simulink model "BANSHEE"  (Simulink 8.1)
settings: Solver=ode1  StartTime=0.0  StopTime=inf  FixedStep=Ts  MaxStep=1e-3  RelTol=1e-3
PostLoadFcn:
  | BANSHEE_init;
InitFcn:
  | BANSHEE_init;
values from neighbouring files (symbols this model uses):
  F1 = xlsread('F1_relay_banshee.xlsx')    [relay_settings_init.m]
  F2 = xlsread('F2_relay_banshee.xlsx')    [relay_settings_init.m]
  F3 = xlsread('F3_relay_banshee.xlsx')    [relay_settings_init.m]
  Ts = 100E-6    (= 0.0001)    [BANSHEE_init.m]    (also in Ghost_init.m)
undefined symbols (not defined in the file or in its folder): Banshee_HWCtrl_IOs, Banshee_SEL751_Woodward_lib, DMS_slave_lib, DMSCommands, fdesignblkfcn, Feeder1_lib, Feeder2_lib, Feeder3_lib, gcbh, generic_ethernet_cb, Hydride, Left, Metal, Nickel, relay_housing_lib, SM_UtilityService, SS_F1_RELAY_HOUSING, SS_F2_RELAY_HOUSING, SS_F3_RELAY_HOUSING, SS_Feeder1, SS_Feeder2, SS_Feeder3, TestSeq_slave_lib, TestSequenceCommands, type, utility_service_lib, V
libraries: powerlib x64, cables_lib x54, breaker_lib x52, rtio_generic_modbus x46, relay_modbus_lib x42, rtio_opalrt_op5142ex1 x37, transformer_lib x29, simulink x26, rteventslib x26, rtlab x24, Load_lib x20, ssn_lib x18
(part 6 of 8)

== system BANSHEE/SM_UtilityService/Banshee_HWCtrl_IOs/Woodward Inputs ==
  note: Copyright (c) 2016 Massachusetts Institute of Technology
      | Permission is hereby granted, free of charge, to any person obtaining a copy of this software and associated documentation files (the "Software"), to deal
      | in the Software without restriction, including without limitation the rights to use, copy, modify, merge, publish, distribute, sublicense, and/or sell copies of the
      | Software, and to permit persons to whom the Software is furnished to do so, subject to the following conditions:
      |
      | THE SOFTWARE IS PROVIDED "AS IS", WITHOUT WARRANTY OF ANY KIND, EXPRESS OR IMPLIED, INCLUDING BUT NOT LIMITED TO THE
      | WARRANTIES OF MERCHANTABILITY, FITNESS FOR A PARTICULAR PURPOSE AND NONINFRINGEMENT. IN NO EVENT SHALL THE AUTHORS
      | OR COPYRIGHT HOLDERS BE LIABLE FOR ANY CLAIM, DAMAGES OR OTHER LIABILITY, WHETHER IN AN ACTION OF CONTRACT, TORT OR
      | OTHERWISE, ARISING FROM, OUT OF OR IN CONNECTION WITH THE SOFTWARE OR THE USE OR OTHER DEALINGS IN THE SOFTWARE
  note: GR1 A AOUT (CH00-15)
  note: All signals should be scaled accordingly prior connecting to this block
  Generator1_Voltage : Inport
  Generator1_Current : Inport  Port=2
  Mains1_Voltage : Inport  Port=3
  Mains1_Current : Inport  Port=4
  MPU1_speed : Inport  Port=5
  Generator2_Voltage : Inport  Port=6
  Generator2_Current : Inport  Port=7
  Mains2_Voltage : Inport  Port=8
  Mains2_Current : Inport  Port=9
  MPU2_speed : Inport  Port=10
  AnalogOut : rtio_opalrt_common/AnalogOut  CtrlName='OpCtrl'  portNb=1  FcnNos=Slot 1 Module A Subsection 1  size=16  maxcount=8  count=8  numchan=8  israngeinput=off  voltagerange=[-16 ... 16]  slot=0  side=0  mismatch=0  slotside=Slot_1_Module_A
      settings: AttributesFormatString=%<CtrlName>
  AnalogOut1 : rtio_opalrt_common/AnalogOut  CtrlName='OpCtrl'  portNb=2  FcnNos=Slot 1 Module A Subsection 2  size=16  maxcount=8  count=8  numchan=8  israngeinput=off  voltagerange=[-16 ... 16]  slot=0  side=0  mismatch=0  slotside=Slot_1_Module_A
      settings: AttributesFormatString=%<CtrlName>
  AnalogOut2 : rtio_opalrt_common/AnalogOut  CtrlName='OpCtrl'  portNb=3  FcnNos=Slot 2 Module A Subsection 1  size=16  maxcount=8  count=8  numchan=8  israngeinput=off  voltagerange=[-16 ... 16]  slot=1  side=0  mismatch=0  slotside=Slot_2_Module_A
      settings: AttributesFormatString=%<CtrlName>
  AnalogOut3 : rtio_opalrt_common/AnalogOut  CtrlName='OpCtrl'  portNb=4  FcnNos=Slot 2 Module A Subsection 2  size=16  maxcount=8  count=8  numchan=8  israngeinput=off  voltagerange=[-16 ... 16]  slot=1  side=0  mismatch=0  slotside=Slot_2_Module_A
      settings: AttributesFormatString=%<CtrlName>
  Demux : Demux  Outputs=2
  Demux{1..5,7..9} (8 alike) : Demux  Outputs=3
  Demux6 : Demux  Outputs=2
  Mux{,1,3..4} (4 alike) : Mux  Inputs=8
  Mux2 : Mux  Inputs=2
  Mux5 : Mux  Inputs=2
  Terminator{,1..3} (4 alike) : Terminator
  wires:
  Mains1_Voltage/1 -> Demux2/1
  Generator1_Voltage/1 -> Demux1/1
  Mux2/1 -> Demux/1
  Mux1/1 -> Mux2/2
  Mux/1 -> Mux2/1
  Demux/2 -> AnalogOut1/1
  Demux/1 -> AnalogOut/1
  AnalogOut1/1 -> Terminator1/1
  AnalogOut/1 -> Terminator/1
  Demux1/1 -> Mux/1
  Demux1/2 -> Mux/2
  Demux1/3 -> Mux/3
  Demux2/1 -> Mux/4
  Demux2/2 -> Mux/5
  Demux2/3 -> Mux/6
  MPU1_speed/1 -> Mux1/5
  Demux4/1 -> Mux/7
  Demux4/2 -> Mux/8
  Demux4/3 -> Mux1/1
  Demux5/1 -> Mux1/2
  Demux5/2 -> Mux1/3
  Demux5/3 -> Mux1/4
  Mux5/1 -> Demux6/1
  Mux4/1 -> Mux5/2
  Mux3/1 -> Mux5/1
  Demux6/2 -> AnalogOut3/1
  Demux6/1 -> AnalogOut2/1
  AnalogOut3/1 -> Terminator3/1
  AnalogOut2/1 -> Terminator2/1
  Generator1_Current/1 -> Demux3/1
  Demux3/1 -> Mux3/2
  Demux3/2 -> Mux3/3
  Demux3/3 -> Mux3/4
  Mains1_Current/1 -> Demux7/1
  Demux7/1 -> Mux3/1
  Mains2_Voltage/1 -> Demux5/1
  Generator2_Voltage/1 -> Demux4/1
  MPU2_speed/1 -> Mux1/6
  Mains2_Current/1 -> Demux8/1
  Demux8/1 -> Mux3/5
  Generator2_Current/1 -> Demux9/1
  Demux9/1 -> Mux3/6
  Demux9/2 -> Mux3/7
  Demux9/3 -> Mux3/8

== system BANSHEE/SM_UtilityService/Banshee_HWCtrl_IOs/Woodward Outputs - Diesel - Gen2 ==
  note: Copyright (c) 2016 Massachusetts Institute of Technology
      | Permission is hereby granted, free of charge, to any person obtaining a copy of this software and associated documentation files (the "Software"), to deal
      | in the Software without restriction, including without limitation the rights to use, copy, modify, merge, publish, distribute, sublicense, and/or sell copies of the
      | Software, and to permit persons to whom the Software is furnished to do so, subject to the following conditions:
      |
      | THE SOFTWARE IS PROVIDED "AS IS", WITHOUT WARRANTY OF ANY KIND, EXPRESS OR IMPLIED, INCLUDING BUT NOT LIMITED TO THE
      | WARRANTIES OF MERCHANTABILITY, FITNESS FOR A PARTICULAR PURPOSE AND NONINFRINGEMENT. IN NO EVENT SHALL THE AUTHORS
      | OR COPYRIGHT HOLDERS BE LIABLE FOR ANY CLAIM, DAMAGES OR OTHER LIABILITY, WHETHER IN AN ACTION OF CONTRACT, TORT OR
      | OTHERWISE, ARISING FROM, OUT OF OR IN CONNECTION WITH THE SOFTWARE OR THE USE OR OTHER DEALINGS IN THE SOFTWARE
  Gen2 MCB Status : Inport
  WoodwardBias : Inport  Port=2
  Bus Creator1 : BusCreator  Inputs=1
  DIO - Gr3 : Subsystem
  DIO - Woodward : Subsystem
  DOUT type config : Subsystem
  Woodward Primary Inputs - Gen2 : Subsystem
  Digital Inputs : Outport
  Gen2 Gov and AVR : Outport  Port=2
  Gen2 Fuel Enable : Outport  Port=3
  Gen2 GCB : Outport  Port=4
  Gen2 MCB : Outport  Port=5
  wires:
  Bus Creator1/1 -> Digital Inputs/1
  DIO - Woodward/1(DIn1) -> DIO - Gr3/1(Dout)
  DIO - Gr3/1(DIn) -> Bus Creator1/1, DIO - Woodward/1(Din_Wood)  "DIN"
  Woodward Primary Inputs - Gen2/1(Gen2 Gov and AVR) -> Gen2 Gov and AVR/1
  DIO - Woodward/3(Gen2 GCB) -> Gen2 GCB/1
  DIO - Woodward/2(Gen2 Fuel Enable) -> Gen2 Fuel Enable/1
  DIO - Woodward/4(Gen2 MCB) -> Gen2 MCB/1
  Gen2 MCB Status/1 -> DIO - Woodward/2(Gen2 MCB Status)
  WoodwardBias/1 -> Woodward Primary Inputs - Gen2/1(WoodwardBias)

== system BANSHEE/SM_UtilityService/Banshee_HWCtrl_IOs/Woodward Outputs - NGCHP - Gen1 ==
  note: Copyright (c) 2016 Massachusetts Institute of Technology
      | Permission is hereby granted, free of charge, to any person obtaining a copy of this software and associated documentation files (the "Software"), to deal
      | in the Software without restriction, including without limitation the rights to use, copy, modify, merge, publish, distribute, sublicense, and/or sell copies of the
      | Software, and to permit persons to whom the Software is furnished to do so, subject to the following conditions:
      |
      | THE SOFTWARE IS PROVIDED "AS IS", WITHOUT WARRANTY OF ANY KIND, EXPRESS OR IMPLIED, INCLUDING BUT NOT LIMITED TO THE
      | WARRANTIES OF MERCHANTABILITY, FITNESS FOR A PARTICULAR PURPOSE AND NONINFRINGEMENT. IN NO EVENT SHALL THE AUTHORS
      | OR COPYRIGHT HOLDERS BE LIABLE FOR ANY CLAIM, DAMAGES OR OTHER LIABILITY, WHETHER IN AN ACTION OF CONTRACT, TORT OR
      | OTHERWISE, ARISING FROM, OUT OF OR IN CONNECTION WITH THE SOFTWARE OR THE USE OR OTHER DEALINGS IN THE SOFTWARE
  Gen1 MCB Status : Inport
  WoodwardBias : Inport  Port=2
  Bus Creator1 : BusCreator  Inputs=1
  DIO - Gr3 : Subsystem
  DIO - Woodward : Subsystem
  DOUT type config : Subsystem
  Woodward Primary Inputs - Gen1 : Subsystem
  Digital Inputs : Outport
  Gen1 Gov and AVR : Outport  Port=2
  Gen1 Fuel Enable : Outport  Port=3
  Gen1 GCB : Outport  Port=4
  Gen1 MCB : Outport  Port=5
  wires:
  DIO - Woodward/4(DIn1) -> DIO - Gr3/1(Dout)
  DIO - Gr3/1(DIn) -> DIO - Woodward/1(Din_Wood), Bus Creator1/1  "DIN"
  Bus Creator1/1 -> Digital Inputs/1
  Woodward Primary Inputs - Gen1/1(Gen1 Gov and AVR) -> Gen1 Gov and AVR/1
  WoodwardBias/1 -> Woodward Primary Inputs - Gen1/1(WoodwardBias)
  DIO - Woodward/2(Gen1 GCB) -> Gen1 GCB/1
  DIO - Woodward/3(Gen1 MCB) -> Gen1 MCB/1
  DIO - Woodward/1(Gen1 Fuel Enable) -> Gen1 Fuel Enable/1
  Gen1 MCB Status/1 -> DIO - Woodward/2(Gen1 MCB Status)

== system BANSHEE/SM_UtilityService/DataSet_Diesel_CHP_PCCs/Status ==
  SEL751 : Inport
  CBX03 : Inport  Port=2
  GCB : Inport  Port=3
  Data Type Conversion{,1..3} (4 alike) : DataTypeConversion
  Gain : Gain  Gain=2
  Gain1 : Gain  Gain=4
  Sum : Sum  Inputs=+++
  o : Outport
  wires:
  GCB/1 -> Data Type Conversion2/1
  CBX03/1 -> Data Type Conversion1/1
  SEL751/1 -> Data Type Conversion/1
  Gain/1 -> Sum/2
  Gain1/1 -> Sum/3
  Sum/1 -> Data Type Conversion3/1
  Data Type Conversion/1 -> Sum/1
  Data Type Conversion1/1 -> Gain/1
  Data Type Conversion2/1 -> Gain1/1
  Data Type Conversion3/1 -> o/1

== system BANSHEE/SM_UtilityService/DataSet_Diesel_CHP_PCCs/Status1 ==
  SEL751 : Inport
  CBX03 : Inport  Port=2
  GCB : Inport  Port=3
  Data Type Conversion{,1..3} (4 alike) : DataTypeConversion
  Gain : Gain  Gain=2
  Gain1 : Gain  Gain=4
  Sum : Sum  Inputs=+++
  o : Outport
  wires:
  GCB/1 -> Data Type Conversion2/1
  CBX03/1 -> Data Type Conversion1/1
  SEL751/1 -> Data Type Conversion/1
  Gain/1 -> Sum/2
  Gain1/1 -> Sum/3
  Sum/1 -> Data Type Conversion3/1
  Data Type Conversion/1 -> Sum/1
  Data Type Conversion1/1 -> Gain/1
  Data Type Conversion2/1 -> Gain1/1
  Data Type Conversion3/1 -> o/1

== system BANSHEE/SM_UtilityService/Number of seconds of recording/Increment ==
  Trigger : TriggerPort
  Increment : Constant
  Memory : Memory  InheritSampleTime=on
  Sum : Sum  Inputs=|++
  Out1 : Outport
  wires:
  Increment/1 -> Sum/2
  Memory/1 -> Sum/1
  Sum/1 -> Memory/1, Out1/1

== system BANSHEE/SM_UtilityService/Number of seconds of recording1/Increment ==
  Trigger : TriggerPort
  Increment : Constant
  Memory : Memory  InheritSampleTime=on
  Sum : Sum  Inputs=|++
  Out1 : Outport
  wires:
  Increment/1 -> Sum/2
  Memory/1 -> Sum/1
  Sum/1 -> Memory/1, Out1/1

== system BANSHEE/SM_UtilityService/selected_Irms_a/rms_a ==
  i : Inport
  Demux1 : Demux  Outputs=3
  RMS_Calculator : RMS_lib/RMS_Calculator  Ts=Ts
  Terminator8 : Terminator
  Terminator9 : Terminator
  o : Outport
  wires:
  i/1 -> Demux1/1
  RMS_Calculator/1 -> o/1
  Demux1/1 -> RMS_Calculator/1
  Demux1/2 -> Terminator8/1
  Demux1/3 -> Terminator9/1

== system BANSHEE/SM_UtilityService/selected_Irms_a/rms_a1 ==
  i : Inport
  Demux1 : Demux  Outputs=3
  RMS_Calculator : RMS_lib/RMS_Calculator  Ts=Ts
  Terminator8 : Terminator
  Terminator9 : Terminator
  o : Outport
  wires:
  i/1 -> Demux1/1
  RMS_Calculator/1 -> o/1
  Demux1/1 -> RMS_Calculator/1
  Demux1/2 -> Terminator8/1
  Demux1/3 -> Terminator9/1

== system BANSHEE/SM_UtilityService/selected_Irms_a/rms_a2 ==
  i : Inport
  Demux1 : Demux  Outputs=3
  RMS_Calculator : RMS_lib/RMS_Calculator  Ts=Ts
  Terminator8 : Terminator
  Terminator9 : Terminator
  o : Outport
  wires:
  i/1 -> Demux1/1
  RMS_Calculator/1 -> o/1
  Demux1/1 -> RMS_Calculator/1
  Demux1/2 -> Terminator8/1
  Demux1/3 -> Terminator9/1

== system BANSHEE/SM_UtilityService/selected_Irms_a/rms_a3 ==
  i : Inport
  Demux1 : Demux  Outputs=3
  RMS_Calculator : RMS_lib/RMS_Calculator  Ts=Ts
  Terminator8 : Terminator
  Terminator9 : Terminator
  o : Outport
  wires:
  i/1 -> Demux1/1
  RMS_Calculator/1 -> o/1
  Demux1/1 -> RMS_Calculator/1
  Demux1/2 -> Terminator8/1
  Demux1/3 -> Terminator9/1

== system BANSHEE/SM_UtilityService/selected_Irms_a/rms_a4 ==
  i : Inport
  Demux1 : Demux  Outputs=3
  RMS_Calculator : RMS_lib/RMS_Calculator  Ts=Ts
  Terminator8 : Terminator
  Terminator9 : Terminator
  o : Outport
  wires:
  i/1 -> Demux1/1
  RMS_Calculator/1 -> o/1
  Demux1/1 -> RMS_Calculator/1
  Demux1/2 -> Terminator8/1
  Demux1/3 -> Terminator9/1

== system BANSHEE/SM_UtilityService/selected_Irms_a/rms_a5 ==
  i : Inport
  Demux1 : Demux  Outputs=3
  RMS_Calculator : RMS_lib/RMS_Calculator  Ts=Ts
  Terminator8 : Terminator
  Terminator9 : Terminator
  o : Outport
  wires:
  i/1 -> Demux1/1
  RMS_Calculator/1 -> o/1
  Demux1/1 -> RMS_Calculator/1
  Demux1/2 -> Terminator8/1
  Demux1/3 -> Terminator9/1

== system BANSHEE/SM_UtilityService/selected_Irms_a/rms_a6 ==
  i : Inport
  Demux1 : Demux  Outputs=3
  RMS_Calculator : RMS_lib/RMS_Calculator  Ts=Ts
  Terminator8 : Terminator
  Terminator9 : Terminator
  o : Outport
  wires:
  i/1 -> Demux1/1
  RMS_Calculator/1 -> o/1
  Demux1/1 -> RMS_Calculator/1
  Demux1/2 -> Terminator8/1
  Demux1/3 -> Terminator9/1

== system BANSHEE/SM_UtilityService/selected_Irms_a/rms_a7 ==
  i : Inport
  Demux1 : Demux  Outputs=3
  RMS_Calculator : RMS_lib/RMS_Calculator  Ts=Ts
  Terminator8 : Terminator
  Terminator9 : Terminator
  o : Outport
  wires:
  i/1 -> Demux1/1
  RMS_Calculator/1 -> o/1
  Demux1/1 -> RMS_Calculator/1
  Demux1/2 -> Terminator8/1
  Demux1/3 -> Terminator9/1

== system BANSHEE/SM_UtilityService/selected_Irms_a/rms_a8 ==
  i : Inport
  Demux1 : Demux  Outputs=3
  RMS_Calculator : RMS_lib/RMS_Calculator  Ts=Ts
  Terminator8 : Terminator
  Terminator9 : Terminator
  o : Outport
  wires:
  i/1 -> Demux1/1
  RMS_Calculator/1 -> o/1
  Demux1/1 -> RMS_Calculator/1
  Demux1/2 -> Terminator8/1
  Demux1/3 -> Terminator9/1

== system BANSHEE/SM_UtilityService/selected_Irms_a/rms_a9 ==
  i : Inport
  Demux1 : Demux  Outputs=3
  RMS_Calculator : RMS_lib/RMS_Calculator  Ts=Ts
  Terminator8 : Terminator
  Terminator9 : Terminator
  o : Outport
  wires:
  i/1 -> Demux1/1
  RMS_Calculator/1 -> o/1
  Demux1/1 -> RMS_Calculator/1
  Demux1/2 -> Terminator8/1
  Demux1/3 -> Terminator9/1

== system BANSHEE/SS_F3_RELAY_HOUSING/Banshee UDP Data - Formatted Packets/Ethernet communication interface ==
  note: Ethernet communication interface example model
  Data trigger : Inport
  Data to send : Inport  Port=2
  AsyncEthernetCtrl : S-Function  InitFcn=generic_ethernet_cb('initfcn');  FunctionName=sfun_gen_async_ctrl  Parameters=ctrl_id, nbr_to_remote_endpoint, type_to_remote_endpoint,nbr_from_remote_endpoint,type_from_remote_endpoint,protocol,tcp_mode, port, offset_to_remote_endpoint,offset_from_remote_endpoint,swap_tx,swap_rx,0,nic_name,remote_ip,'','','','','','','','','','',exe_name,0  EnableBusSupport=off  mask(AsyncEthernetCtrl){ctrl_id=1, nbr_to_remote_endpoint=342, type_to_remote_endpoint=INT32, offset_to_remote_endpoint=0, nbr_from_remote_endpoint=4, type_from_remote_endpoint=DOUBLE, offset_from_remote_endpoint=0, nic_name=eth0, protocol=UDP, tcp_mode=Server, port=7200, remote_ip=255.255.255.255, exe_name=AsyncEthernet, swap_tx=off, swap_rx=off}
      mask prompts: ctrl_id "Controller ID"; nbr_to_remote_endpoint "Number of data to send"; type_to_remote_endpoint "Type of data to send"; offset_to_remote_endpoint "Byte offset of transmission buffer"; nbr_from_remote_endpoint "Number of data expected to be received"; type_from_remote_endpoint "Type of data expected to be received"; offset_from_remote_endpoint "Byte offset of reception buffer"; nic_name "Network interface name"; tcp_mode "TCP mode"; remote_ip "Remote IP address"; exe_name "Name of the executable"; swap_tx "Swap data endianness before transmission"; swap_rx "Swap data endianness after reception"
      mask help: Generic asynchronous process configuration block
      mask Help: eval('rtlab_help(''opasyncgenctrl'');');
      mask TypeOptions type_to_remote_endpoint: UINT8 | INT8 | UINT16 | INT16 | UINT32 | INT32 | FLOAT | DOUBLE
      mask TypeOptions type_from_remote_endpoint: UINT8 | INT8 | UINT16 | INT16 | UINT32 | INT32 | FLOAT | DOUBLE
      mask TypeOptions protocol: UDP | TCP
      mask TypeOptions tcp_mode: Client | Server
      mask Display: disp(sprintf('\nEthernet communication \ninterface controller\n'))
  B-width : SignalSpecification  Dimensions=nbr_from_remote_endpoint
  Constant : Constant  Value=1000
  Logo : opal_lib/Logo1  vide=[]
  Mux : Mux  Inputs=2
  OpAsyncRecv : rtlab/Communication/Asynchronous/OpAsyncRecv  ctl_id=ctrl_id  recv_id=ctrl_id  enable_param=off  fp1=1  fp2=2  fp3=3  fp4=4  fp5=5  sp1=string1  sp2=string2  sp3=string3  sp4=string4  sp5=string5
  OpAsyncSend : rtlab/Communication/Asynchronous/OpAsyncSend  ctl_id=ctrl_id  send_id=ctrl_id  mode=DONT_NEED_REPLY  enable_param=off  fp1=1  fp2=2  fp3=3  fp4=4  fp5=5  sp1=string1  sp2=string2  sp3=string3  sp4=string4  sp5=string5
  Terminator : Terminator
  Data received : Outport
  Status : Outport  Port=2
  wires:
  Data to send/1 -> OpAsyncSend/2
  Data trigger/1 -> OpAsyncSend/1
  OpAsyncSend/1 -> Mux/1
  OpAsyncRecv/1 -> Mux/2
  Mux/1 -> Status/1
  Constant/1 -> OpAsyncRecv/1
  OpAsyncRecv/2 -> Terminator/1
  OpAsyncRecv/3 -> B-width/1
  B-width/1 -> Data received/1

== system BANSHEE/SS_PV_BESS/EPC/BMS_Modbus ==
  BESS_MS : Inport
  Bus Selector : BusSelector  OutputSignals=Battery_Meas.SOC (%),Battery_Meas.Current (A),Battery_Meas.Voltage (V),BESS_MX1.cb_ms.Status,BESS_MX1.VRMSLL,BESS_MX1.Freq,BESS_MX1.kw,BESS_MX1.kvar
  Gain : Gain  Gain=100
  Gain1 : Gain  Gain=100
  Modbus device6 : rtio_generic_modbus/Modbus device  conf_name=EPC_BMS_cfg.opal  conf_name_mask=EPC_BMS_cfg.xls  sample_time=Ts
  Mux : Mux  Inputs=8
  wires:
  Bus Selector/7 -> Mux/7  "<kw>"
  Bus Selector/5 -> Mux/5  "<VRMSLL>"
  Bus Selector/1 -> Gain/1  "<SOC (%)>"
  Bus Selector/6 -> Gain1/1  "<Freq>"
  Bus Selector/8 -> Mux/8  "<kvar>"
  BESS_MS/1 -> Bus Selector/1
  Gain/1 -> Mux/1
  Bus Selector/3 -> Mux/3  "<Voltage (V)>"
  Bus Selector/2 -> Mux/2  "<Current (A)>"
  Bus Selector/4 -> Mux/4  "<Status>"
  Gain1/1 -> Mux/6
  Mux/1 -> Modbus device6/1

== system BANSHEE/SS_PV_BESS/EPC/Contactors1 ==
  note: with 10ohm resistor
  note: changed to 1000
      | to slow down the time
  Precharge : Inport
  Main Contactor : Inport  Port=2
  Brk_Battery : powerlib/Power Electronics/Ideal Switch  Ron=0.001  Lon=0  IC=0  Rs=1e6  Cs=inf  Measurements=on
  Brk_Precharge : powerlib/Power Electronics/Ideal Switch  Ron=1  Lon=0  IC=0  Rs=1e6  Cs=inf  Measurements=on
  DC+ Source : PMIOPort  Port=1  Side=Right
  DC+ Bus : PMIOPort  Port=2  Side=Left
  DC- Source : PMIOPort  Port=3  Side=Left
  DC- Bus : PMIOPort  Port=4  Side=Right
  wires:
  Precharge/1 -> Brk_Precharge/1
  Main Contactor/1 -> Brk_Battery/1
  connections:
  Brk_Battery/LConn1 -- DC+ Bus/RConn1 -- Brk_Precharge/LConn1
  Brk_Battery/RConn1 -- DC+ Source/RConn1 -- Brk_Precharge/RConn1
  DC- Bus/RConn1 -- DC- Source/RConn1

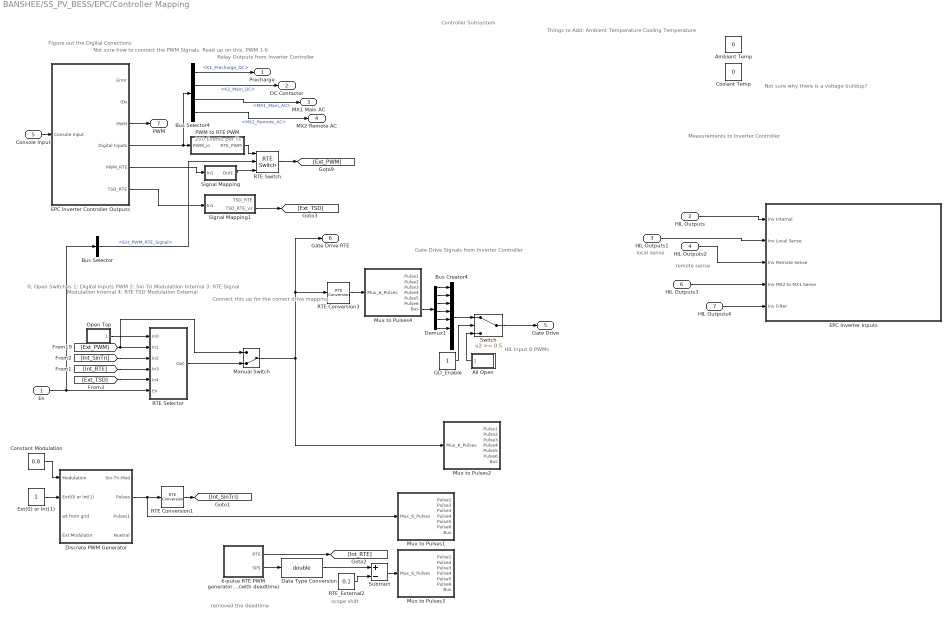
== system BANSHEE/SS_PV_BESS/EPC/Controller Mapping ==
  note: Controller Subsystem
  note: Gate Drive Signals from
      | Inverter Controller
  note: Relay Outputs from
      | Inverter Controller
  note: Measurements to
      | Inverter Controller
  note: Not sure why there is a voltage buildup?
  note: Things to Add:
      | Ambient Temperature
      | Cooling Temperature
  note: HIL Input
      | 8 PWMs
  note: local sense
  note: remote sense
  note: Not sure how to connect
      | the PWM Signals.
      | Read up on this.
      | PWM 1-6
  note: Figure out the
      | Digital Conections
  note: removed the deadtime
  note: scope shift
  note: 0; Open Switches
      | 1: Digital Inputs PWM
      | 2: Sin Tri Modulatiion Internal
      | 3: RTE Signal Modulation Internal
      | 4: RTE TSD Modulation External
  note: 200 Events per Ts
  note: Connect this
      | up for the
      | correct drive
      | mapping.
  En : Inport
  HIL Outputs : Inport  Port=2
  HIL Outputs1 : Inport  Port=3
  HIL Outputs2 : Inport  Port=4
  Console Input : Inport  Port=5
  HIL Outputs3 : Inport  Port=6
  HIL Outputs4 : Inport  Port=7
  6-pulse RTE PWM generator (with deadtime) : Subsystem  Tag=RTEcontrol_s38shd7k88  AncestorBlock=|  mask(3-phase RT-Event Discrete PWM Generator){GeneratorMode=3-arm  bridge (6 pulses), Fc=5000, Ts=Ts, mIndex=0.9, Freq=60, Phase=0, Tdead=0}
      | artemis/Tools /Rt-Event 
      | control blocks/6-pulse RTE
      | PWM generator
      | (with deadtime)
      mask prompts: GeneratorMode "Generator Mode"; Fc "Carrier frequency (Hz):"; Ts "Sample time:"; mIndex "Modulation index  (0<m<1) :"; Freq "Frequency of output voltage (Hz)"; Phase "Phase of output voltage (degrees)"; Tdead "Deadtime (s)"
      mask help:
      | This  block generates RT-Event pulses for 3-phase discrete time compensated  carrier-based PWM (Pulse Width Modulation), self-commutated IGBTs,GTOs or FETs bridges in ARTEMIS-RTE.
      |
      | RT-Event pulses are pair of signals that contain the logical value of the switch {on.off} and a timing value used in ARTEMIS-RTE to compensate for in-step switching actions.
      | PSB pulses consist of the logicla part only.
      |
      | Pulses 1,3 and 5 are respectively for the upper switches of the first,second and third arm. Pulses 2,4 and 6 are for the lower switches.
      mask init:
      | set_param(gcb,'LinkStatus','inactive');
      | if Freq==0
      |     Phase=90;
      | end
      |     Internal_Phase=[0 -2*pi/3 2*pi/3];
      |     Signal_PortWidth=3;
      |     Select1_Elements=[1 4 2 5 3 6];
      |     Select1_PortWidth=6;
      |    Select3_Elements=[1 2 3 4 5 6];
      |    Select3_PortWidth=12;
      mask TypeOptions GeneratorMode: 3-arm  bridge (6 pulses)
      mask Display: plot(0,0,100,100,[60,57,57,56,56,53,53,50,50,47,47,41,41,38,38,35,35,32,32,31,31,25,25,24,24,22,22,19,19,16,16,11,11,8,8,5,5,3,3,2,2,0],[20,20,80,80,20,20,80,80,20,20,80,80,20,20,80,80,20,20,80,80,20,20,80,80,20,20,80,80,20,20,80,80,20,20,80,80,20,20,80,80,20,20])
  All Open : Subsystem
  Ambient Temp : Constant  Value=0
  Bus Creator4 : BusCreator  Inputs=8
  Bus Selector : BusSelector  OutputSignals=Ext_PWM_RTE_Signal
  Bus Selector4 : BusSelector  OutputSignals=DIN.DI_CH00-07.K1_Precharge_DC,DIN.DI_CH00-07.K2_Main_DC,DIN.DI_CH00-07.MX1_Main_AC,DIN.DI_CH00-07.MX2_Remote_AC
  Constant Modulation : Constant  Value=0.8
  Coolant Temp : Constant  Value=0
  Data Type Conversion : DataTypeConversion  OutDataTypeStr=double
  Demux1 : Demux  Outputs=6
  Discrete PWM Generator : Subsystem  AncestorBlock=|  DialogController=POWERSYS.PowerSysDialog  mask(Discrete PWM Generator){GeneratorMode=3-arm  bridge (6 pulses), Fc=5000, Ts=Ts, Internal=on, mIndex=0.8, Freq=60, Phase=0}
      | powerlib_extras/Discrete 
      | Control Blocks/Discrete
      | PWM Generator
      mask prompts: GeneratorMode "Generator Mode"; Fc "Carrier frequency (Hz):"; Ts "Sample time:"; Internal "Internal generation of modulating signal(s)"; mIndex "Modulation index  (0<m<1) :"; Freq "Frequency of output voltage (Hz)"; Phase "Phase of output voltage (degrees)"
      mask help:
      | This discrete block generates pulses for carrier-based PWM (Pulse Width Modulation), self-commutated IGBTs,GTOs or FETs bridges.
      |
      | Depending on the number of bridge arms selected in the "Generator Mode" parameter, the block can be used either for single-phase or three-phase PWM control.
      mask init:
      | powericon('psbcallbacks',gcb,'Discrete PWM Generator');
      | if Freq==0
      |     Phase=90;
      | end
      | switch GeneratorMode
      | case 1,
      |     Internal_Phase=0;
      |    Signal_PortWidth=1;
      |    Select1_Elements=[1 2];
      |    Select1_PortWidth=2;
      |    Select3_Elements=[1 2];
      |    Select3_PortWidth=4;
      | case 2,
      |     Internal_Phase=0;
      |     Signal_PortWidth=1;
      |     Select1_Elements=[1 2];
      |     Select1_PortWidth=2;
      |     Select3_Elements=[1 2 3 4];
      |     Select3_PortWidth=4;
      | case 3,
      |     Internal_Phase=[0 -2*pi/3 2*pi/3];
      |     Signal_PortWidth=3;
      |     Select1_Elements=[1 4 2 5 3 6];
      |     Select1_PortWidth=6;
      |    Select3_Elements=[1 2 3 4 5 6];
      |    Select3_PortWidth=12;
      | case 4,
      |     Internal_Phase=[0 -2*pi/3 2*pi/3];
      |     Signal_PortWidth=3;
      |     Select1_Elements=[1 4 2 5 3 6];
      |     Select1_PortWidth=6;
      |    Select3_Elements=[1 2 3 4 5 6 7 8 9 10 11 12];
      |    Select3_PortWidth=12;
      | end
      | power_initmask();
      mask Help:
      | The output pulses are a vector (with values=0 or 1). Depending on the selected "Generator Mode", the output vector contains:
      | For a 1-arm  bridge: Two pulses. Pulse 1 is for the upper switch and pulse 2 is for the lower switch.
      | For a 2-arm  bridge: Four pulses. Pulses 1 and 3 are respectively for the upper switches of the first and second arm. Pulses 2 and 4 are for the lower switches.
      | For a 3-arm  bridge: Six pulses. Pulses 1,3 and 5 are respectively for the upper switches of the first,second and third arm. Pulses 2,4 and 6 are for the lower switches.
      | For double 3-arm bridges: Twelve pulses.The first six pulses (pulses 1 to 6) must be sent to the first 3-arm bridge and the last six (pulses 7 to 12) to the second 3-arm bridge.
      | 
      | By selecting "Internal generation" you can can control the modulation index m, frequency and phase of the output voltage  from the internal parameters (m, Freq and Phase). Otherwise, external signals are used for pulse generation. The width of the input vector must be 1 for single phase bridges ( 1-arm or 2-arm)  and 3 for 3-phase bridges  (single or double bridge).
      mask TypeOptions GeneratorMode: 1-arm  bridge (2 pulses) | 2-arm  bridge (4 pulses) | 3-arm  bridge (6 pulses) | Double 3-arm  bridges (12 pulses)
      mask Callback Internal: %powericon('psbcallbacks',gcb,'Discrete PWM Generator',[]);
      mask Display: disp('')
  EPC Inverter Controller Outputs : Subsystem
  EPC Inverter Inputs : Subsystem
  Ext(0) or Int(1) : Constant
  GD_Enable : Constant
  Manual Switch : ManualSwitch  CurrentSetting=0
  Mux to Pulses1 : Subsystem
  Mux to Pulses2 : Subsystem
  Mux to Pulses3 : Subsystem
  Mux to Pulses4 : Subsystem
  Open Top : Subsystem
  PWM to RTE PWM : Subsystem
  RTE Conversion1 : rteventslib/Signal Attributes/RTE Conversion  inputdatatype=Double  outputdatatype=RTE Boolean  compensation=Enabled  nbMaxEvents=4  sampleTime=Ts
  RTE Conversion3 : rteventslib/Signal Attributes/RTE Conversion  inputdatatype=RTE Boolean  outputdatatype=Double  compensation=Enabled  nbMaxEvents=4  sampleTime=Ts
  RTE Selector : Subsystem
  RTE Switch : rteventslib/Signal Routing/RTE Switch  switchType=u2 = Double; u1 u3 = RTE Boolean  criteria=u2 >= Threshold  threshold=0.5  interpolate=on  nbMaxEvents=4
  RTE_External2 : Constant  Value=0.1
  Signal Mapping : Subsystem
  Signal Mapping1 : Subsystem
  Subtract : Sum  Inputs=+-
  Switch : Switch  Threshold=0.5
  Precharge : Outport
  DC Contactor : Outport  Port=2
  MX1 Main AC : Outport  Port=3
  MX2 Remote AC : Outport  Port=4
  Gate Drive : Outport  Port=5
  Gate Drive RTE : Outport  Port=6
  PWM : Outport  Port=7
  wires:
  Signal Mapping1/2(TSD_RTE_v2) -> [Ext_TSD]
  Demux1/3 -> Bus Creator4/3
  Demux1/5 -> Bus Creator4/5
  GD_Enable/1 -> Switch/2
  Demux1/1 -> Bus Creator4/1
  Demux1/2 -> Bus Creator4/2
  Bus Creator4/1 -> Switch/1
  All Open/1(Pulses8) -> Switch/3
  Demux1/4 -> Bus Creator4/4
  Demux1/6 -> Bus Creator4/6
  HIL Outputs/1 -> EPC Inverter Inputs/1(Inv Internal)
  Console Input/1 -> EPC Inverter Controller Outputs/1(Console Input)
  Constant Modulation/1 -> Discrete PWM Generator/1(Modulation)
  Ext(0) or Int(1)/1 -> Discrete PWM Generator/2(Ext(0) or Int(1))
  6-pulse RTE PWM generator (with deadtime)/1(RTE) -> [Int_RTE]
  RTE Conversion3/1 -> Mux to Pulses4/1(Mux_6_Pulses)
  Mux to Pulses4/7(Bus) -> Demux1/1
  Switch/1 -> Gate Drive/1
  6-pulse RTE PWM generator (with deadtime)/2(SPS) -> Data Type Conversion/1
  Data Type Conversion/1 -> Subtract/1
  RTE_External2/1 -> Subtract/2
  Subtract/1 -> Mux to Pulses3/1(Mux_6_Pulses)
  Bus Selector4/2 -> DC Contactor/1  "<K2_Main_DC>"
  Bus Selector4/1 -> Precharge/1  "<K1_Precharge_DC>"
  EPC Inverter Controller Outputs/3(PWM) -> PWM/1
  RTE Conversion1/1 -> [Int_SinTri]
  Discrete PWM Generator/2(Pulses) -> RTE Conversion1/1, Mux to Pulses1/1(Mux_6_Pulses)
  [Int_SinTri] -> RTE Selector/3(In2)
  Open Top/1(Pulses6) -> RTE Selector/1(In0)
  [Int_RTE] -> RTE Selector/4(In3)
  En/1 -> RTE Selector/6(En), Bus Selector/1
  [Ext_PWM] -> Manual Switch/1, RTE Selector/2(In1)
  RTE Selector/1(Out) -> Manual Switch/2
  Manual Switch/1 -> Mux to Pulses2/1(Mux_6_Pulses), RTE Conversion3/1, Gate Drive RTE/1
  EPC Inverter Controller Outputs/5(PWM_RTE) -> Signal Mapping/1(In1)
  Signal Mapping/1(Out1) -> RTE Switch/3
  RTE Switch/1 -> [Ext_PWM]
  PWM to RTE PWM/1(RTE_PWM) -> RTE Switch/1
  Bus Selector/1 -> RTE Switch/2  "<Ext_PWM_RTE_Signal>"
  EPC Inverter Controller Outputs/4(Digital Inputs) -> Bus Selector4/1, PWM to RTE PWM/1(PWM_in)
  EPC Inverter Controller Outputs/6(TSD_RTE) -> Signal Mapping1/1(In1)
  [Ext_TSD] -> RTE Selector/5(In4)
  HIL Outputs1/1 -> EPC Inverter Inputs/2(Inv Local Sense)
  HIL Outputs2/1 -> EPC Inverter Inputs/3(Inv Remote Sense)
  Bus Selector4/3 -> MX1 Main AC/1  "<MX1_Main_AC>"
  Bus Selector4/4 -> MX2 Remote AC/1  "<MX2_Remote_AC>"
  HIL Outputs3/1 -> EPC Inverter Inputs/4(Inv MX2 to MX1 Sense)
  HIL Outputs4/1 -> EPC Inverter Inputs/5(Inv Filter)

== system BANSHEE/SS_PV_BESS/EPC/Inverter_Batt_RTE ==
  note: What does the maximum number of events mean for RTE?
      | What should this be set to?
  note: 1 e-4
      | 1.1 Vf
      | 10 Events
  note: Now 200 Events
  Gate_Drives_RTE : Inport
  Bus Creator1 : BusCreator  Inputs=7
  DC_Bus : powerlib/Elements/Parallel RLC Branch  LConnTagsString=a  RConnTagsString=__new0  BranchType=RC  Resistance=20e3  Inductance=1e-3  SetiL0=off  InitialCurrent=0  Capacitance=2*(925e-6)  Setx0=on  InitialVoltage=0  Measurements=None
  Inv1 : powerlib/Measurements/Current Measurement  PhasorSimulation=off  OutputType=Complex  PSBequivalent=0
  Inv2 : powerlib/Measurements/Current Measurement  PhasorSimulation=off  OutputType=Complex  PSBequivalent=0
  Inv3 : powerlib/Measurements/Current Measurement  PhasorSimulation=off  OutputType=Complex  PSBequivalent=0
  Inv_DC1 : powerlib/Measurements/Current Measurement  PhasorSimulation=off  OutputType=Complex  PSBequivalent=0
  Inv_DC2 : powerlib/Measurements/Current Measurement  PhasorSimulation=off  OutputType=Complex  PSBequivalent=0
  TSB_hiZ snubber_free (contains 6 real diode) : Subsystem
      mask Display: plot(0,0,100,100,[34,34],[60,90],[34,34],[20,50],[60,50],[60,60],[55,59,50,55],[60,50,50,60],[55,55,34],[50,34,34],[34,55,55],[75,75,60],[29,34],[57,50],[23,23,26,23,23,13],[55,51,55,58,55,55])
  V_DClink_1 : powerlib/Measurements/Voltage Measurement  PhasorSimulation=off  OutputType=Complex  PSBequivalent=0
  V_DClink_2 : powerlib/Measurements/Voltage Measurement  PhasorSimulation=off  OutputType=Complex  PSBequivalent=0
  Inv_1 : PMIOPort  Port=1  Side=Left
  Inv_2 : PMIOPort  Port=2  Side=Left
  Inv_3 : PMIOPort  Port=3  Side=Left
  DC+ : PMIOPort  Port=4  Side=Right
  DC- : PMIOPort  Port=5  Side=Right
  m : Outport
  wires:
  Gate_Drives_RTE/1 -> TSB_hiZ snubber_free (contains 6 real diode)/1(g)
  Inv3/1 -> [Inv_Ph3_W_Iout]
  Inv1/1 -> [Inv_Ph1_U_Iout]
  Inv2/1 -> [Inv_Ph2_V_Iout]
  V_DClink_1/1 -> [Inv_Vdc1]
  V_DClink_2/1 -> [Inv_Vdc2]
  Bus Creator1/1 -> m/1
  [Inv_Ph1_U_Iout] -> Bus Creator1/1  "Inv_1"
  [Inv_Ph2_V_Iout] -> Bus Creator1/2  "Inv_2"
  [Inv_Ph3_W_Iout] -> Bus Creator1/3  "Inv_3"
  [Inv_Idc1] -> Bus Creator1/4  "Inv_Idc1"
  [Inv_Idc2] -> Bus Creator1/5  "Inv_Idc2"
  [Inv_Vdc1] -> Bus Creator1/6  "Inv_Vdc1"
  [Inv_Vdc2] -> Bus Creator1/7  "Inv_Vdc2"
  Inv_DC1/1 -> [Inv_Idc1]
  Inv_DC2/1 -> [Inv_Idc2]
  connections:
  Inv_DC1/RConn1 -- TSB_hiZ snubber_free (contains 6 real diode)/RConn1
  TSB_hiZ snubber_free (contains 6 real diode)/LConn1 -- Inv1/RConn1
  TSB_hiZ snubber_free (contains 6 real diode)/LConn2 -- Inv2/RConn1
  TSB_hiZ snubber_free (contains 6 real diode)/LConn3 -- Inv3/RConn1
  DC_Bus/LConn1 -- Inv_DC2/RConn1 -- V_DClink_2/LConn1 -- Inv_DC1/LConn1 -- V_DClink_1/LConn1
  DC+/RConn1 -- Inv_DC2/LConn1
  Inv_1/RConn1 -- Inv1/LConn1
  Inv_2/RConn1 -- Inv2/LConn1
  Inv_3/RConn1 -- Inv3/LConn1
  DC-/RConn1 -- DC_Bus/RConn1 -- V_DClink_2/LConn2 -- TSB_hiZ snubber_free (contains 6 real diode)/RConn2 -- V_DClink_1/LConn2

== system BANSHEE/SS_PV_BESS/EPC/LCL Filter 200kW1 ==
  note: High Resistor:
      | 10e6 ohms
      | Numerical Stability
  note: Create a three wire version that removes the Inv 4 port and 4 nuetral.
      | There is a reistor in parallel with the capacitor for the discharge voltage at shutoff.
  Bleed_R1 : powerlib/Elements/Series RLC Branch  LConnTagsString=__new0  RConnTagsString=__new0  BranchType=R  Resistance=filter_cap_bleed_res  Inductance=1e-3  SetiL0=off  InitialCurrent=0  Capacitance=filter_cap  Setx0=on  InitialVoltage=0  Measurements=None
  Bleed_R2 : powerlib/Elements/Series RLC Branch  LConnTagsString=__new0  RConnTagsString=__new0  BranchType=R  Resistance=filter_cap_bleed_res  Inductance=1e-3  SetiL0=off  InitialCurrent=0  Capacitance=filter_cap  Setx0=on  InitialVoltage=0  Measurements=None
  Bleed_R3 : powerlib/Elements/Series RLC Branch  LConnTagsString=__new0  RConnTagsString=__new0  BranchType=R  Resistance=filter_cap_bleed_res  Inductance=1e-3  SetiL0=off  InitialCurrent=0  Capacitance=filter_cap  Setx0=on  InitialVoltage=0  Measurements=None
  Capacitor_L1 : powerlib/Elements/Series RLC Branch  LConnTagsString=__new0  RConnTagsString=__new0  BranchType=RC  Resistance=filter_cap_res  Inductance=1e-3  SetiL0=off  InitialCurrent=0  Capacitance=filter_cap  Setx0=on  InitialVoltage=0  Measurements=None
  Capacitor_L2 : powerlib/Elements/Series RLC Branch  LConnTagsString=__new0  RConnTagsString=__new0  BranchType=RC  Resistance=filter_cap_res  Inductance=1e-3  SetiL0=off  InitialCurrent=0  Capacitance=filter_cap  Setx0=on  InitialVoltage=0  Measurements=None
  Capacitor_L3 : powerlib/Elements/Series RLC Branch  LConnTagsString=__new0  RConnTagsString=__new0  BranchType=RC  Resistance=filter_cap_res  Inductance=1e-3  SetiL0=off  InitialCurrent=0  Capacitance=filter_cap  Setx0=on  InitialVoltage=0  Measurements=None
  Inductor_Inv1 : powerlib/Elements/Series RLC Branch  LConnTagsString=__new0  RConnTagsString=__new0  BranchType=RL  Resistance=filter_inv_res  Inductance=filter_inv_ind  SetiL0=off  InitialCurrent=0  Capacitance=1e-6  Setx0=off  InitialVoltage=0  Measurements=None
  Inductor_Inv2 : powerlib/Elements/Series RLC Branch  LConnTagsString=__new0  RConnTagsString=__new0  BranchType=RL  Resistance=filter_inv_res  Inductance=filter_inv_ind  SetiL0=off  InitialCurrent=0  Capacitance=1e-6  Setx0=off  InitialVoltage=0  Measurements=None
  Inductor_Inv3 : powerlib/Elements/Series RLC Branch  LConnTagsString=__new0  RConnTagsString=__new0  BranchType=RL  Resistance=filter_inv_res  Inductance=filter_inv_ind  SetiL0=off  InitialCurrent=0  Capacitance=1e-6  Setx0=off  InitialVoltage=0  Measurements=None
  Inductor_Inv4 : powerlib/Elements/Series RLC Branch  LConnTagsString=__new0  RConnTagsString=__new0  BranchType=L  Resistance=1  Inductance=filter_inv_ind  SetiL0=off  InitialCurrent=0  Capacitance=1e-6  Setx0=off  InitialVoltage=0  Measurements=None
  Inductor_L1 : powerlib/Elements/Series RLC Branch  LConnTagsString=__new0  RConnTagsString=__new0  BranchType=RL  Resistance=filter_line_res  Inductance=filter_line_ind  SetiL0=off  InitialCurrent=0  Capacitance=1e-6  Setx0=off  InitialVoltage=0  Measurements=None
  Inductor_L2 : powerlib/Elements/Series RLC Branch  LConnTagsString=__new0  RConnTagsString=__new0  BranchType=RL  Resistance=filter_line_res  Inductance=filter_line_ind  SetiL0=off  InitialCurrent=0  Capacitance=1e-6  Setx0=off  InitialVoltage=0  Measurements=None
  Inductor_L3 : powerlib/Elements/Series RLC Branch  LConnTagsString=__new0  RConnTagsString=__new0  BranchType=RL  Resistance=filter_line_res  Inductance=filter_line_ind  SetiL0=off  InitialCurrent=0  Capacitance=1e-6  Setx0=off  InitialVoltage=0  Measurements=None
  Three-Phase Series RLC Branch : powerlib/Elements/Three-Phase Series RLC Branch  LConnTagsString=A|B|C  RConnTagsString=A|B|C  BranchType=R  Resistance=1e6  Inductance=1e-3  Capacitance=1e-6  Measurements=None
  A : PMIOPort  Port=1  Side=Left
  B : PMIOPort  Port=2  Side=Left
  C : PMIOPort  Port=3  Side=Left
  N : PMIOPort  Port=4  Side=Left
  Inv_1 : PMIOPort  Port=5  Side=Right  mask{filter_line_ind=[], filter_cap=0, filter_inv_ind=0}
      mask prompts: filter_line_ind "Line Filter Inductor (H)"; filter_cap "Filter Capacitor (F)"; filter_inv_ind "Inverter Filter Inductor (H)"
  Inv_2 : PMIOPort  Port=6  Side=Right
  Inv_3 : PMIOPort  Port=7  Side=Right
  Inv_4 : PMIOPort  Port=8  Side=Right
  connections:
  Inductor_L1/RConn1 -- Inductor_Inv1/LConn1 -- Capacitor_L1/LConn1 -- Bleed_R1/LConn1
  Inv_1/RConn1 -- Inductor_Inv1/RConn1
  A/RConn1 -- Inductor_L1/LConn1
  Inductor_L2/RConn1 -- Inductor_Inv2/LConn1 -- Capacitor_L2/LConn1 -- Bleed_R2/LConn1
  Inv_2/RConn1 -- Inductor_Inv2/RConn1
  B/RConn1 -- Inductor_L2/LConn1
  Inductor_L3/RConn1 -- Inductor_Inv3/LConn1 -- Capacitor_L3/LConn1 -- Bleed_R3/LConn1
  Inv_3/RConn1 -- Inductor_Inv3/RConn1
  C/RConn1 -- Inductor_L3/LConn1
  N/RConn1 -- Capacitor_L1/RConn1 -- Bleed_R1/RConn1 -- Capacitor_L2/RConn1 -- Bleed_R2/RConn1 -- Capacitor_L3/RConn1 -- Bleed_R3/RConn1 -- Inductor_Inv4/LConn1
  Inv_4/RConn1 -- Inductor_Inv4/RConn1

== system BANSHEE/SC_ctrl/EPC Inverter/16TSDIn/16 TSDOut GR3/Din/Dout ch16-23 ==
  Bus Creator3 : BusCreator  Inputs=8
  times17 : Constant  Value=[0.05 0.15 0.25 0.35]
  times18 : Constant  Value=[0.1 0.2 0.3 0.4]
  times19 : Constant  Value=[0.15 0.25 0.35 0.45]
  times20 : Constant  Value=[0.2 0.3 0.4 0.5]
  times21 : Constant  Value=[0.25 0.35 0.45 0.55]
  times22 : Constant  Value=[0.3 0.4 0.5 0.6]
  times23 : Constant  Value=[0.3 0.4 0.5 0.6]
  times24 : Constant  Value=[0 0.1 0.2 0.3]
  Out1 : Outport
  wires:
  times24/1 -> Bus Creator3/1  "times17"
  times17/1 -> Bus Creator3/2  "times18"
  times18/1 -> Bus Creator3/3  "times19"
  times19/1 -> Bus Creator3/4  "times20"
  times20/1 -> Bus Creator3/5  "times21"
  times21/1 -> Bus Creator3/6  "times22"
  times22/1 -> Bus Creator3/7  "times23"
  times23/1 -> Bus Creator3/8  "times24"
  Bus Creator3/1 -> Out1/1

== system BANSHEE/SC_ctrl/EPC Inverter/16TSDIn/16 TSDOut GR3/Din/Dout ch24-31 ==
  Bus Creator4 : BusCreator  Inputs=8
  times25 : Constant  Value=[0.05 0.15 0.25 0.35]
  times26 : Constant  Value=[0.1 0.2 0.3 0.4]
  times27 : Constant  Value=[0.15 0.25 0.35 0.45]
  times28 : Constant  Value=[0.2 0.3 0.4 0.5]
  times29 : Constant  Value=[0.25 0.35 0.45 0.55]
  times30 : Constant  Value=[0.3 0.4 0.5 0.6]
  times31 : Constant  Value=[0.3 0.4 0.5 0.6]
  times32 : Constant  Value=[0 0.1 0.2 0.3]
  Out1 : Outport
  wires:
  times32/1 -> Bus Creator4/1  "times25"
  times25/1 -> Bus Creator4/2  "times26"
  times26/1 -> Bus Creator4/3  "times27"
  times27/1 -> Bus Creator4/4  "times28"
  times28/1 -> Bus Creator4/5  "times29"
  times29/1 -> Bus Creator4/6  "times30"
  times30/1 -> Bus Creator4/7  "times31"
  times31/1 -> Bus Creator4/8  "times32"
  Bus Creator4/1 -> Out1/1

== system BANSHEE/SC_ctrl/EPC Inverter/16TSDIn/16 TSDOut GR3/Dout state ctrl ==
  Bus Creator : BusCreator  Inputs=2
  Dout_CH16_CH23 : Subsystem
  Dout_CH24_CH31 : Subsystem
  Event State OUT : Outport
  wires:
  Bus Creator/1 -> Event State OUT/1
  Dout_CH16_CH23/1(Dout_CH8_CH15) -> Bus Creator/1  "CH16-23"
  Dout_CH24_CH31/1(Dout_CH8_CH15) -> Bus Creator/2  "CH24-31"

== system BANSHEE/SM_UtilityService/Banshee_HWCtrl_IOs/SEL751_DigitalAnalog_IO_OpBlocks/F1 ==
  Substation : Inport
  Feeder : Inport  Port=2
  DTT : Inport  Port=3
  TS_SQ : Inport  Port=4
  Logical Operator : Logic  AllPortsSameDT=off  OutDataTypeStr=boolean
  Logical Operator1 : Logic  Operator=OR  Inputs=3  AllPortsSameDT=off  OutDataTypeStr=boolean
  Logical Operator2 : Logic  Operator=OR  AllPortsSameDT=off  OutDataTypeStr=boolean
  Logical Operator3 : Logic  Operator=NOT  AllPortsSameDT=off  OutDataTypeStr=boolean
  Logical Operator5 : Logic  Operator=NOT  AllPortsSameDT=off  OutDataTypeStr=boolean
  trip : Outport
  wires:
  DTT/1 -> Logical Operator2/1
  Feeder/1 -> Logical Operator5/1
  Logical Operator5/1 -> Logical Operator1/2
  Substation/1 -> Logical Operator3/1
  Logical Operator3/1 -> Logical Operator1/1
  Logical Operator1/1 -> Logical Operator/1
  Logical Operator/1 -> trip/1
  Logical Operator2/1 -> Logical Operator/2
  TS_SQ/1 -> Logical Operator1/3, Logical Operator2/2

== system BANSHEE/SM_UtilityService/Banshee_HWCtrl_IOs/SEL751_DigitalAnalog_IO_OpBlocks/F2 ==
  Substation : Inport
  Feeder : Inport  Port=2
  DTT : Inport  Port=3
  TS_SQ : Inport  Port=4
  Logical Operator : Logic  AllPortsSameDT=off  OutDataTypeStr=boolean
  Logical Operator1 : Logic  Operator=OR  Inputs=3  AllPortsSameDT=off  OutDataTypeStr=boolean
  Logical Operator2 : Logic  Operator=OR  AllPortsSameDT=off  OutDataTypeStr=boolean
  Logical Operator3 : Logic  Operator=NOT  AllPortsSameDT=off  OutDataTypeStr=boolean
  Logical Operator5 : Logic  Operator=NOT  AllPortsSameDT=off  OutDataTypeStr=boolean
  trip : Outport
  wires:
  DTT/1 -> Logical Operator2/1
  Feeder/1 -> Logical Operator5/1
  Logical Operator5/1 -> Logical Operator1/2
  Substation/1 -> Logical Operator3/1
  Logical Operator3/1 -> Logical Operator1/1
  Logical Operator1/1 -> Logical Operator/1
  Logical Operator/1 -> trip/1
  Logical Operator2/1 -> Logical Operator/2
  TS_SQ/1 -> Logical Operator1/3, Logical Operator2/2

== system BANSHEE/SM_UtilityService/Banshee_HWCtrl_IOs/SEL751_DigitalAnalog_IO_OpBlocks/F3 ==
  Substation : Inport
  Feeder : Inport  Port=2
  DTT : Inport  Port=3
  TS_SQ : Inport  Port=4
  Logical Operator : Logic  AllPortsSameDT=off  OutDataTypeStr=boolean
  Logical Operator1 : Logic  Operator=OR  Inputs=3  AllPortsSameDT=off  OutDataTypeStr=boolean
  Logical Operator2 : Logic  Operator=OR  AllPortsSameDT=off  OutDataTypeStr=boolean
  Logical Operator3 : Logic  Operator=NOT  AllPortsSameDT=off  OutDataTypeStr=boolean
  Logical Operator5 : Logic  Operator=NOT  AllPortsSameDT=off  OutDataTypeStr=boolean
  trip : Outport
  wires:
  DTT/1 -> Logical Operator2/1
  Feeder/1 -> Logical Operator5/1
  Logical Operator5/1 -> Logical Operator1/2
  Substation/1 -> Logical Operator3/1
  Logical Operator3/1 -> Logical Operator1/1
  Logical Operator1/1 -> Logical Operator/1
  Logical Operator/1 -> trip/1
  Logical Operator2/1 -> Logical Operator/2
  TS_SQ/1 -> Logical Operator1/3, Logical Operator2/2

== system BANSHEE/SM_UtilityService/Banshee_HWCtrl_IOs/Woodward Outputs - Diesel - Gen2/DIO - Gr3 ==
  Dout : Inport
  Bus Creator : BusCreator  Inputs=1
  Bus Selector1 : BusSelector  OutputSignals=DI_CH08-15  OutputAsBus=on
  Conditioning1 : Subsystem
  DigitalIn1 : rtio_opalrt_common/DigitalIn  CtrlName='OpCtrl'  portNb=6  FcnNos=Slot 3 Module A Subsection 2  size=1  maxcount=8  count=8  sampleTime=0  numchan=8
      settings: AttributesFormatString=%<CtrlName>
  DigitalOut1 : rtio_opalrt_common/DigitalOut  CtrlName='OpCtrl'  portNb=6  FcnNos=Slot 3 Module B Subsection 2  size=1  maxcount=8  count=8  numchan=8
      settings: AttributesFormatString=%<CtrlName>
  Terminator1 : Terminator
  Terminator6 : Terminator
  DIn : Outport
  wires:
  DigitalOut1/1 -> Terminator1/1
  Dout/1 -> Bus Selector1/1
  Bus Selector1/1 -> DigitalOut1/1
  DigitalIn1/2 -> Terminator6/1
  DigitalIn1/1 -> Conditioning1/1(In1)  "DI_CH08-15"
  Bus Creator/1 -> DIn/1
  Conditioning1/1(Out1) -> Bus Creator/1

== system BANSHEE/SM_UtilityService/Banshee_HWCtrl_IOs/Woodward Outputs - Diesel - Gen2/DIO - Woodward ==
  note: Copyright (c) 2016 Massachusetts Institute of Technology
      | Permission is hereby granted, free of charge, to any person obtaining a copy of this software and associated documentation files (the "Software"), to deal
      | in the Software without restriction, including without limitation the rights to use, copy, modify, merge, publish, distribute, sublicense, and/or sell copies of the
      | Software, and to permit persons to whom the Software is furnished to do so, subject to the following conditions:
      |
      | THE SOFTWARE IS PROVIDED "AS IS", WITHOUT WARRANTY OF ANY KIND, EXPRESS OR IMPLIED, INCLUDING BUT NOT LIMITED TO THE
      | WARRANTIES OF MERCHANTABILITY, FITNESS FOR A PARTICULAR PURPOSE AND NONINFRINGEMENT. IN NO EVENT SHALL THE AUTHORS
      | OR COPYRIGHT HOLDERS BE LIABLE FOR ANY CLAIM, DAMAGES OR OTHER LIABILITY, WHETHER IN AN ACTION OF CONTRACT, TORT OR
      | OTHERWISE, ARISING FROM, OUT OF OR IN CONNECTION WITH THE SOFTWARE OR THE USE OR OTHER DEALINGS IN THE SOFTWARE
  note: Ch08-11
  note: These are the inputs to
      | the HIL Outputs.
  Din_Wood : Inport
  Gen2 MCB Status : Inport  Port=2
  Add2 : Sum
  Add3 : Sum
  Bus Creator : BusCreator  Inputs=1
  Bus Selector5 : BusSelector  OutputSignals=DI_CH08-15.Gen2_Starter,DI_CH08-15.Gen2_Fuel
  Bus Selector6 : BusSelector  OutputSignals=DI_CH08-15.Gen2_Open_GCB,DI_CH08-15.Gen2_Close_GCB,DI_CH08-15.Gen2_Open_MCB,DI_CH08-15.Gen2_Close_MCB
  Compare To Zero{7..8,10..12} (5 alike) : simulink/Logic and Bit Operations/Compare To Zero  relop=>  OutDataTypeStr=boolean
  Compare To Zero13 : simulink/Logic and Bit Operations/Compare To Zero  relop=<=  OutDataTypeStr=boolean
  Constant : Constant  Value=0
  Constant1 : Constant
  Constant3 : Constant
  Constant4 : Constant
  Constant5 : Constant  Value=0
  Data Type Conversion{,1..3} (4 alike) : DataTypeConversion  OutDataTypeStr=double
  Logical Operator1 : Logic  Operator=NOT  AllPortsSameDT=off  OutDataTypeStr=boolean
  Mux1 : Mux  Inputs=8
  S-R Flip-Flop3 : simulink_extras/Flip Flops/S-R Flip-Flop  initial_condition=1
  S-R Flip-Flop4 : simulink_extras/Flip Flops/S-R Flip-Flop  initial_condition=1
  S-R Flip-Flop5 : simulink_extras/Flip Flops/S-R Flip-Flop  initial_condition=0
  Switch5 : Switch  Threshold=0.5
  Terminator : Terminator
  Terminator1 : Terminator
  DIn1 : Outport
  Gen2 Fuel Enable : Outport  Port=2
  Gen2 GCB : Outport  Port=3
  Gen2 MCB : Outport  Port=4
  wires:
  Constant1/1 -> Mux1/1  "Estop"
  Data Type Conversion3/1 -> Mux1/8
  Data Type Conversion2/1 -> Mux1/7
  Data Type Conversion1/1 -> Mux1/6
  Constant/1 -> Mux1/4, Mux1/3, Mux1/2
  S-R Flip-Flop5/2 -> Terminator1/1
  S-R Flip-Flop4/2 -> Terminator/1
  Din_Wood/1 -> Bus Selector5/1, Bus Selector6/1
  Bus Creator/1 -> DIn1/1
  Mux1/1 -> Bus Creator/1  "DI_CH08-15"
  S-R Flip-Flop3/1 -> Data Type Conversion1/1, Add2/1
  Bus Selector6/1 -> Compare To Zero7/1  "<Gen2_Open_GCB>"
  Compare To Zero7/1 -> S-R Flip-Flop3/1
  Compare To Zero8/1 -> S-R Flip-Flop3/2
  Bus Selector6/4 -> Compare To Zero11/1  "<Gen2_Close_MCB>"
  Compare To Zero11/1 -> S-R Flip-Flop4/2
  Bus Selector6/3 -> Compare To Zero10/1  "<Gen2_Open_MCB>"
  Compare To Zero10/1 -> S-R Flip-Flop4/1
  Bus Selector6/2 -> Compare To Zero8/1  "<Gen2_Close_GCB>"
  S-R Flip-Flop4/1 -> Add3/2
  Add2/1 -> Gen2 GCB/1
  Add3/1 -> Gen2 MCB/1
  Constant3/1 -> Add2/2, Add3/1
  Bus Selector5/1 -> Compare To Zero12/1  "<Gen2_Starter>"
  Bus Selector5/2 -> Compare To Zero13/1  "<Gen2_Fuel>"
  S-R Flip-Flop5/1 -> Switch5/2
  Compare To Zero12/1 -> S-R Flip-Flop5/1
  Constant5/1 -> Switch5/3
  Constant4/1 -> Switch5/1
  Compare To Zero13/1 -> S-R Flip-Flop5/2
  Switch5/1 -> Gen2 Fuel Enable/1
  Gen2 MCB Status/1 -> Logical Operator1/1, Data Type Conversion2/1
  S-R Flip-Flop3/2 -> Data Type Conversion3/1
  Logical Operator1/1 -> Data Type Conversion/1
  Data Type Conversion/1 -> Mux1/5

== system BANSHEE/SM_UtilityService/Banshee_HWCtrl_IOs/Woodward Outputs - Diesel - Gen2/DOUT type config ==
  note: The Constants are used to select Digital Output type:
      | - 0: Time-Stamped Digital Output
      | - 1: Pulse-Width Modulated DIgital Output
  DataIn Send1 : rtio_opalrt_common/DataIn Send  CtrlName='OpCtrl'  FcnNos=12  width=1  portType=double  checkVersion=off  expectedId=0  expectedVersion=0  opComp=>=
      settings: AttributesFormatString=%<CtrlName>
  Subsection 4 DOUT type : Constant
  Terminator1 : Terminator
  wires:
  Subsection 4 DOUT type/1 -> DataIn Send1/1
  DataIn Send1/1 -> Terminator1/1
